simulink model "onofgalo2"  (R2024b)
settings: Solver=VariableStepAuto  StartTime=0.0  StopTime=120  RelTol=1e-3
libraries: opcualib x2, sldrtlib x1
settings Model: Creator=PROBOOK  LastModifiedBy=PROBOOK

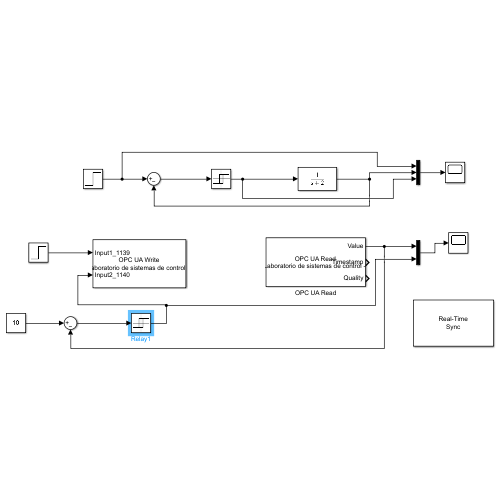
[thumbnail: Simulink's stored preview of the top-level diagram]
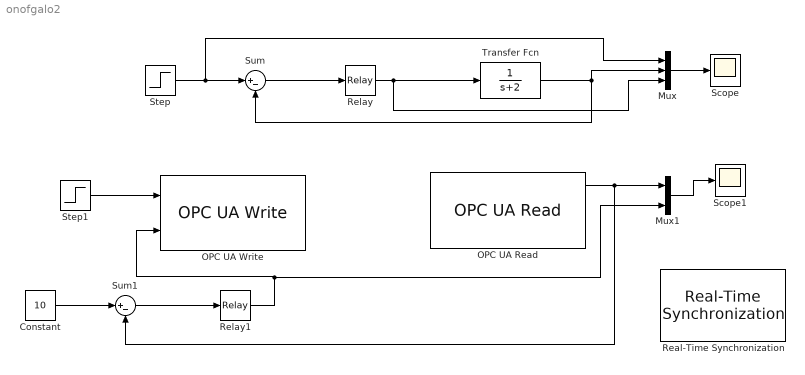
== system onofgalo2 ==
  Constant : Constant  Value=10
  Mux : Mux  Inputs=3
  Mux1 : Mux  Inputs=2
  OPC UA Read : opcualib/OPC UA Read  SelectedServer=UCuenca - Laboratorio de sistemas de control - open62541  ServerList=UCuenca - Laboratorio de sistemas de control - open62541  NodeList={ '1', 'Output', '1', '1141', '1' }  ShowQualityPort=on  ShowTimestampPort=on  ShowTimestampPortAs=Seconds since start  SampleTime=-1
  OPC UA Write : opcualib/OPC UA Write  SelectedServer=UCuenca - Laboratorio de sistemas de control - open62541  ServerList=UCuenca - Laboratorio de sistemas de control - open62541  SampleTime=-1  NodeList={ '1', 'Input1', '1', '1139', '1'; '2', 'Input2', '1', '1140', '1' }
  Real-Time Synchronization : sldrtlib/Real-Time Synchronization  SampleTime=0.1  MaxMissedTicks=10  ShowMissedTicks=off  YieldWhenWaiting=off
  Relay : Relay  OnSwitchValue=0.1  OffSwitchValue=-0.1  OnOutputValue=10
  Relay1 : Relay  OnSwitchValue=0.1  OffSwitchValue=-0.1  OnOutputValue=0  OffOutputValue=1
  Scope : Scope
  Scope1 : Scope
  Step : Step  Time=10  Before=1  After=2  SampleTime=0
  Step1 : Step  Time=5  After=60  SampleTime=0
  Sum : Sum  Inputs=|+-
  Sum1 : Sum  Inputs=|+-
  Transfer Fcn : TransferFcn  Denominator=[1 2]
  wires:
  Sum/1 -> Relay/1
  Step/1 -> Mux/1, Sum/1
  Mux/1 -> Scope/1
  Transfer Fcn/1 -> Mux/2, Sum/2
  Relay/1 -> Mux/3, Transfer Fcn/1
  Step1/1 -> OPC UA Write/1
  OPC UA Read/1 -> Sum1/2, Mux1/1
  Mux1/1 -> Scope1/1
  Constant/1 -> Sum1/1
  Sum1/1 -> Relay1/1
  Relay1/1 -> Mux1/2, OPC UA Write/2
